simulink model "lab05_4"  (R2018b)
settings: Solver=VariableStepAuto  StartTime=0.0  StopTime=25  RelTol=1e-3
settings Model: Creator=Ivan  LastModifiedBy=Ivan

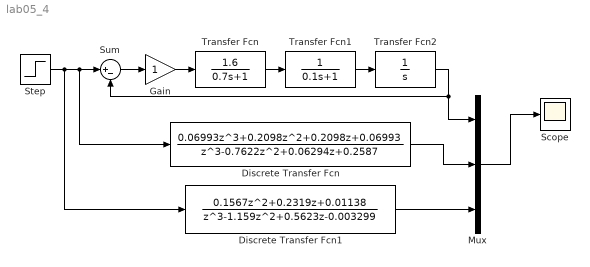
== system lab05_4 ==
  Discrete Transfer Fcn : DiscreteTransferFcn  Numerator=[0.06993 0.2098 0.2098 0.06993]  Denominator=[1 -0.7622 0.06294 0.2587]
  Discrete Transfer Fcn1 : DiscreteTransferFcn  Numerator=[0.1567 0.2319 0.01138]  Denominator=[1 -1.159 0.5623 -0.003299]
  Gain : Gain
  Mux : Mux  Inputs=3
  Scope : Scope
  Step : Step  Before=1  SampleTime=0.5
  Sum : Sum  Inputs=|+-
  Transfer Fcn : TransferFcn  Numerator=[1.6]  Denominator=[0.7 1]
  Transfer Fcn1 : TransferFcn  Denominator=[0.1 1]
  Transfer Fcn2 : TransferFcn  Denominator=[1 0]
  wires:
  Transfer Fcn2/1 -> Sum/2, Mux/1
  Step/1 -> Discrete Transfer Fcn1/1, Discrete Transfer Fcn/1, Sum/1
  Sum/1 -> Gain/1
  Discrete Transfer Fcn/1 -> Mux/2
  Transfer Fcn/1 -> Transfer Fcn1/1
  Gain/1 -> Transfer Fcn/1
  Transfer Fcn1/1 -> Transfer Fcn2/1
  Mux/1 -> Scope/1
  Discrete Transfer Fcn1/1 -> Mux/3
